simulink library "dspwwvlib"  (Simulink 5.1)
values from neighbouring files (symbols this model uses):
  D = var(Noisef)    [lmsxy.m]
  Ts = 1/8000    (= 0.000125)    [dspwwvgen.m]
undefined symbols (not defined in the file or in its folder): b, magnitude
libraries: dspsrcs4 x4, dspsnks4 x2, dspmlti3 x2, dspwin32 x1, dspswit3 x1, dspsigattribs x1, dspindex x1
settings Model: Creator=don  LastModifiedBy=don  ProdHWDeviceType=Microprocessor

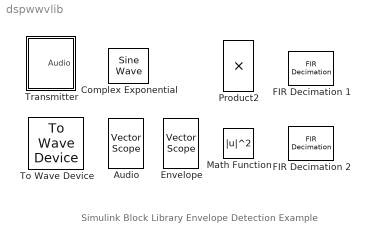
== system dspwwvlib ==
  note: Simulink Block Library
      | Envelope Detection Example
  Audio : dspsnks4/Vector Scope  ScopeProperties=off  Domain=Time  HorizSpan=40  DisplayProperties=off  AxisGrid=on  Memory=off  FrameNumber=on  AxisLegend=off  AxisZoom=off  OpenScopeAtSimStart=on  OpenScopeImmediately=off  FigPos=[430 331 524 241]  AxisProperties=on  XUnits=Hertz  XRange=[0...Fs/2]  InheritXIncr=on  XIncr=1  XLabel=Time  YUnits=dB  YLabel=Amplitude  LineProperties=off
      settings: YMin=-1.1  YMax=1.1
  Complex Exponential : dspsrcs4/Sine Wave  Orientation=down  Amplitude=1  Frequency=100  Phase=0  SampleMode=Discrete  OutComplex=Complex  CompMethod=Table lookup  TableSize=Memory  SampleTime=1/8000  SamplesPerFrame=80  dataType=single  wordLen=16  udDataType=sfix(16)  fracBitsMode=Best precision  numFracBits=14  ResetState=Restart at time zero
      settings: additionalParams=on
  Envelope : dspsnks4/Vector Scope  ScopeProperties=off  Domain=Time  HorizSpan=40  DisplayProperties=off  AxisGrid=on  Memory=off  FrameNumber=on  AxisLegend=off  AxisZoom=off  OpenScopeAtSimStart=on  OpenScopeImmediately=off  FigPos=[426 60 526 225]  AxisProperties=off  XUnits=Hertz  XRange=[0...Fs/2]  InheritXIncr=on  XIncr=1  XLabel=Time  YUnits=dB  YLabel=Amplitude  LineProperties=off
      settings: YMin=-0.1  YMax=0.5
  FIR Decimation 1 : dspmlti3/FIR Decimation  h=fir1(31, 1/40)  D=20  framing=Maintain input frame rate  outputBufInitCond=0  roundingMode=Floor  overflowMode=off
  FIR Decimation 2 : dspmlti3/FIR Decimation  h=fir1(15, 1/8)  D=4  framing=Maintain input frame rate  outputBufInitCond=0  roundingMode=Floor  overflowMode=off
  Math Function : Math  Operator=magnitude^2
  Product2 : Product  SaturateOnIntegerOverflow=on  InputSameDT=on
  To Wave Device : dspwin32/To Wave Device  bufDuration=.25  initDelay=.1  useDefaultDevice=on  enable24Bit=off
  Transmitter : Subsystem

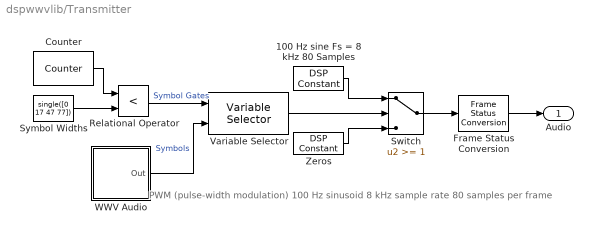
== system dspwwvlib/Transmitter ==
  note: PWM (pulse-width modulation)
      | 100 Hz sinusoid
      | 8 kHz sample rate
      | 80 samples per frame
  100 Hz sine Fs = 8 kHz 80 Samples : dspsrcs4/DSP Constant  Value=single(sin(2*pi*100*(0:79)/8000))  SampleMode=Continuous  discreteOutput=Sample-based (interpret vectors as 1-D)  continuousOutput=Sample-based (interpret vectors as 1-D)  sampTime=1  framePeriod=1  dataType=Inherit from 'Constant value'  wordLen=16  udDataType=sfix(16)  fracBitsMode=Best precision  numFracBits=15  InterpretAs1D=on  Ts=1  FramebasedOutput=off
  Counter : dspswit3/Counter  Direction=Up  CountEvent=Free running  CounterSize=User defined  MaxCount=99  InitialCount=0  Output=Count  HitValue=32  ResetInput=off  SamplesPerFrame=1  Ts=1/100  CntDtype=Single  HitDtype=Logical
  Frame Status Conversion : dspsigattribs/Frame Status Conversion  growRefPort=off  outframe=Frame-based
  Relational Operator : RelationalOperator  Operator=<  InputSameDT=on
  Switch : Switch  Threshold=1  SaturateOnIntegerOverflow=on  InputSameDT=on
  Symbol Widths : Constant  Value=single([0 17 47 77])
  Variable Selector : dspindex/Variable Selector  rowsOrCols=Rows  IdxMode=Variable  Elements=[1 3]  ZerOneIdxMode=Zero-based  errmode=Clip and Warn
  WWV Audio : Subsystem  mask(WWV Audio Synthesizer){outp=Symbols, utc=12.34, ut1=+0.2, day=336, yr=2002, dst=off, dst2=off, leap=on, bufsize=1}
      mask prompts: outp "Output:"; utc "Time (hh.mm):"; ut1 "UT1 Correction ([-0.7, +0.7]):"; day "Day of year:"; yr "Year:"; dst "Daylight Savings"; dst2 "Daylight Savings #2"; leap "Leap second"; bufsize "Samples per frame:"
      mask help: Generate 8 kHz sampled test data in WWV IRIG format.
      mask init:
      | s.utc=utc;s.ut1=ut1;s.day=day;s.yr=yr;
      | s.dst=dst;s.dst2=dst2;s.leap=leap; s.mode=outp;
      | [b,Ts]=dspwwvgen(s);
      | 
      | if strcmp(outp,'Audio'),
      | 
      | x = [.1 .2 .2 .1 .1 NaN .2 .35 .35 .2 .2 NaN .35 .4 .4 .35 .35];
      | y = [.4 .4 .6 .6 .4 NaN .4 .1  .9  .6 .4 NaN .1  .1 .9 .9  .1 ];
      | a=.5;  s=5*pi/180;  t = -s:pi/180:s; x = [x NaN a*cos(t)]; y = [y NaN a*sin(t)+.5];
      | a=.65; s=10*pi/180; t = -s:pi/180:s; x = [x NaN a*cos(t)]; y = [y NaN a*sin(t)+.5];
      | a=.8;  s=20*pi/180; t = -s:pi/180:s; x = [x NaN a*cos(t)]; y = [y NaN a*sin(t)+.5];
      | 
      | else
      | x = [.1 .2 .2 .3 .3 .5 .5 .8 .8 .9];
      | y = [.2 .2 .8 .8 .2 .2 .8 .8 .2 .2];
      | end
      mask Help: Generate 8 kHz sampled test data in WWV IRIG format.
      mask StyleString: popup(Symbols|Audio),edit,edit,edit,edit,checkbox,checkbox,checkbox,edit
      mask Display: plot(x,y)
  Zeros : dspsrcs4/DSP Constant  Value=single(zeros(80,1))  SampleMode=Continuous  discreteOutput=Sample-based (interpret vectors as 1-D)  continuousOutput=Sample-based (interpret vectors as 1-D)  sampTime=1  framePeriod=1  dataType=Inherit from 'Constant value'  wordLen=16  udDataType=sfix(16)  fracBitsMode=Best precision  numFracBits=15  InterpretAs1D=on  Ts=1  FramebasedOutput=off
  Audio : Outport
  wires:
  Frame Status Conversion/1 -> Audio/1
  Relational Operator/1 -> Variable Selector/1  "Symbol Gates"
  Symbol Widths/1 -> Relational Operator/2
  Counter/1 -> Relational Operator/1
  WWV Audio/1(Out) -> Variable Selector/2  "Symbols"
  Variable Selector/1 -> Switch/2
  Switch/1 -> Frame Status Conversion/1
  Zeros/1 -> Switch/3
  100 Hz sine Fs = 8 kHz 80 Samples/1 -> Switch/1

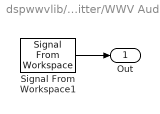
== system dspwwvlib/Transmitter/WWV Audio ==
  Signal From Workspace1 : dspsrcs4/Signal From Workspace  X=int8(b)  Ts=Ts  nsamps=bufsize  OutputAfterFinalValue=Setting to zero
  Out : Outport  InitialOutput=0
  wires:
  Signal From Workspace1/1 -> Out/1
